simulink model "Throttle_Position_Sensors"  (R2022b)
settings: Solver=VariableStepAuto  StartTime=0.0  StopTime=10.0  RelTol=1e-3
settings Model: Creator=yasso  LastModifiedBy=yasso

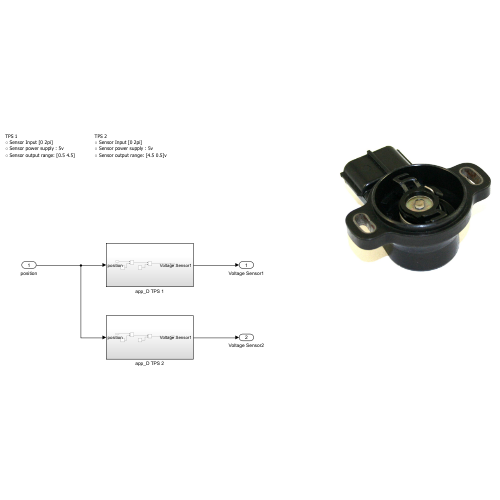
[thumbnail: Simulink's stored preview of the top-level diagram]
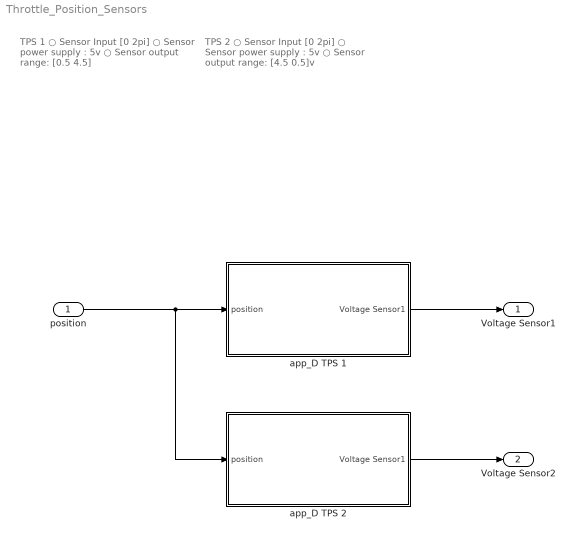
== system Throttle_Position_Sensors ==
  note: TPS 2
      | ○ Sensor Input [0 2pi]
      | ○ Sensor power supply : 5v
      | ○ Sensor output range: [4.5 0.5]v
  note: TPS 1
      | ○ Sensor Input [0 2pi]
      | ○ Sensor power supply : 5v
      | ○ Sensor output range: [0.5 4.5]
  position : Inport
  app_D TPS 1 : Subsystem
  app_D TPS 2 : Subsystem
  Voltage Sensor1 : Outport
  Voltage Sensor2 : Outport  Port=2
  wires:
  app_D TPS 1/1(Voltage Sensor1) -> Voltage Sensor1/1
  app_D TPS 2/1(Voltage Sensor1) -> Voltage Sensor2/1
  position/1 -> app_D TPS 2/1(position), app_D TPS 1/1(position)

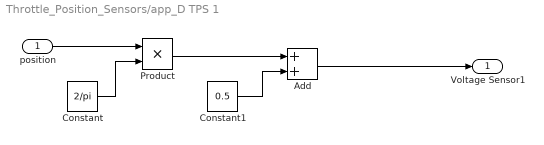
== system Throttle_Position_Sensors/app_D TPS 1 ==
  position : Inport
  Add : Sum
  Constant : Constant  Value=2/pi
  Constant1 : Constant  Value=0.5
  Product : Product
  Voltage Sensor1 : Outport
  wires:
  position/1 -> Product/1
  Constant/1 -> Product/2
  Product/1 -> Add/1
  Constant1/1 -> Add/2
  Add/1 -> Voltage Sensor1/1

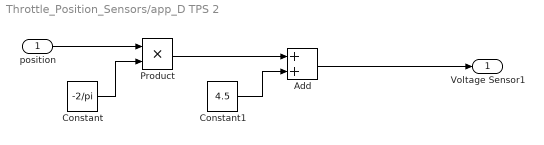
== system Throttle_Position_Sensors/app_D TPS 2 ==
  position : Inport
  Add : Sum
  Constant : Constant  Value=-2/pi
  Constant1 : Constant  Value=4.5
  Product : Product
  Voltage Sensor1 : Outport
  wires:
  Add/1 -> Voltage Sensor1/1
  Constant1/1 -> Add/2
  Product/1 -> Add/1
  Constant/1 -> Product/2
  position/1 -> Product/1
